simulink model "gm_smartCart4_work"  (R2016a)
settings: Solver=FixedStepDiscrete  StartTime=0.0  StopTime=500000  FixedStep=1  RelTol=1e-3
libraries: simulink x103, hdlsllib x73
(part 2 of 3)

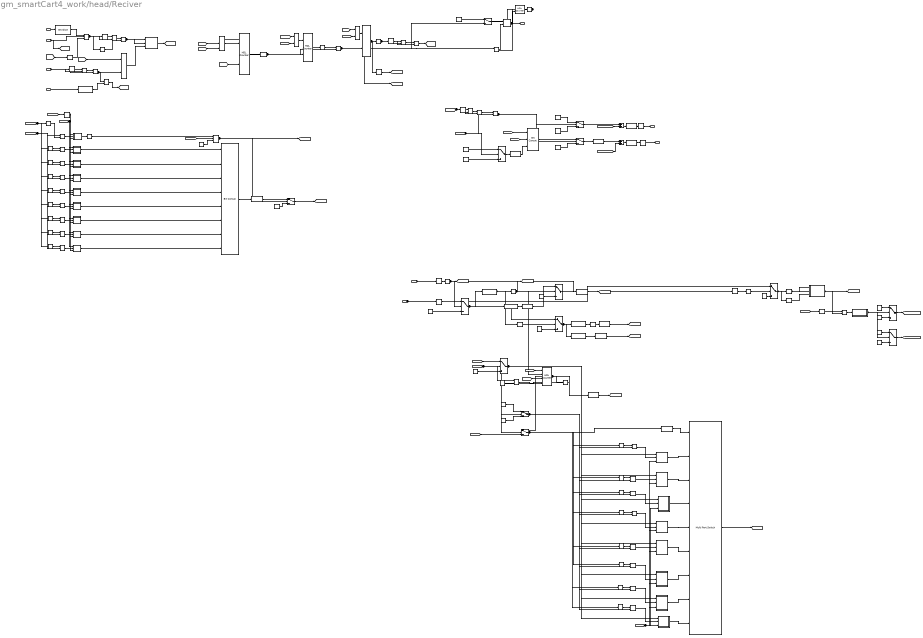
== system gm_smartCart4_work/head/Reciver ==
  note: Схема обнаружение сообщения (1)
  note: cхема управления и синхронизации (2)
  note: Схема формирования отчёта о работе приёмника (4)
  note: Схема связи (5)
  note: Cхема формирования байта и проверка четности
  RST : Inport  OutDataTypeStr=fixdt(1,4,0)  SampleTime=1
  IO : Inport  Port=2  OutDataTypeStr=boolean  SampleTime=1
  STOP : Inport  Port=3  OutDataTypeStr=boolean  SampleTime=1
  adr_IN : Inport  Port=4  OutDataTypeStr=uint8  SampleTime=1
  data_in : Inport  Port=5  OutDataTypeStr=uint32  SampleTime=1
  ON_RECIVER : Inport  Port=6  OutDataTypeStr=boolean  SampleTime=1
  Add : Sum
  Add1 : Sum
  Bit Concat : hdlsllib/HDL Operations/Bit Concat  numInputs=8
  Bit Concat1 : hdlsllib/HDL Operations/Bit Concat  numInputs=3
  Bit Slice1 : hdlsllib/HDL Operations/Bit Slice  lidx=3  ridx=3
  Bit Slice2 : hdlsllib/HDL Operations/Bit Slice  lidx=1  ridx=0
  Bit Slice3 : hdlsllib/HDL Operations/Bit Slice  lidx=7  ridx=2
  Bit Slice4 : hdlsllib/HDL Operations/Bit Slice  lidx=2  ridx=2
  Bit Slice5 : hdlsllib/HDL Operations/Bit Slice  lidx=8  ridx=3
  Compare To Constant{1,3,13,21,31..32} (6 alike) : simulink/Logic and Bit Operations/Compare To Constant  relop===  const=0  OutDataTypeStr=boolean
  Compare To Constant10 : simulink/Logic and Bit Operations/Compare To Constant  relop===  const=7  OutDataTypeStr=boolean
  Compare To Constant11 : simulink/Logic and Bit Operations/Compare To Constant  relop===  const=8  OutDataTypeStr=boolean
  Compare To Constant14 : simulink/Logic and Bit Operations/Compare To Constant  relop===  const=6  OutDataTypeStr=boolean
  Compare To Constant15 : simulink/Logic and Bit Operations/Compare To Constant  relop===  const=7  OutDataTypeStr=boolean
  Compare To Constant{5,16,18,20,22,30} (6 alike) : simulink/Logic and Bit Operations/Compare To Constant  relop===  const=1  OutDataTypeStr=boolean
  Compare To Constant17 : simulink/Logic and Bit Operations/Compare To Constant  relop===  const=200  OutDataTypeStr=boolean
  Compare To Constant19 : simulink/Logic and Bit Operations/Compare To Constant  relop===  const=2  OutDataTypeStr=boolean
  Compare To Constant2 : simulink/Logic and Bit Operations/Compare To Constant  relop===  const=10  OutDataTypeStr=boolean
  Compare To Constant23 : simulink/Logic and Bit Operations/Compare To Constant  relop===  const=2  OutDataTypeStr=boolean
  Compare To Constant24 : simulink/Logic and Bit Operations/Compare To Constant  relop===  const=3  OutDataTypeStr=boolean
  Compare To Constant25 : simulink/Logic and Bit Operations/Compare To Constant  relop===  const=4  OutDataTypeStr=boolean
  Compare To Constant26 : simulink/Logic and Bit Operations/Compare To Constant  relop===  const=5  OutDataTypeStr=boolean
  Compare To Constant27 : simulink/Logic and Bit Operations/Compare To Constant  relop===  const=6  OutDataTypeStr=boolean
  Compare To Constant28 : simulink/Logic and Bit Operations/Compare To Constant  relop===  const=7  OutDataTypeStr=boolean
  Compare To Constant29 : simulink/Logic and Bit Operations/Compare To Constant  relop===  const=5  OutDataTypeStr=boolean
  Compare To Constant4 : simulink/Logic and Bit Operations/Compare To Constant  relop===  const=2604  OutDataTypeStr=boolean
  Compare To Constant6 : simulink/Logic and Bit Operations/Compare To Constant  relop===  const=2  OutDataTypeStr=boolean
  Compare To Constant7 : simulink/Logic and Bit Operations/Compare To Constant  relop===  const=3  OutDataTypeStr=boolean
  Compare To Constant8 : simulink/Logic and Bit Operations/Compare To Constant  relop===  const=4  OutDataTypeStr=boolean
  Compare To Constant9 : simulink/Logic and Bit Operations/Compare To Constant  relop===  const=5  OutDataTypeStr=boolean
  Constant : Constant  Value=0  OutDataTypeStr=uint8
  Constant1 : Constant  Value=0  OutDataTypeStr=uint8
  Constant10 : Constant  Value=0  OutDataTypeStr=boolean  SampleTime=-1
  Constant11 : Constant  Value=0  OutDataTypeStr=boolean
  Constant12 : Constant  Value=0  OutDataTypeStr=uint8
  Constant{3,7,13..15} (5 alike) : Constant  Value=0  OutDataTypeStr=uint32  SampleTime=-1
  Constant16 : Constant  Value=0  OutDataTypeStr=uint8  SampleTime=-1
  Constant17 : Constant  Value=5  OutDataTypeStr=uint8  SampleTime=-1
  Constant18 : Constant  OutDataTypeStr=uint8  SampleTime=-1
  Constant2 : Constant  OutDataTypeStr=uint8
  Constant4 : Constant  Value=2  OutDataTypeStr=fixdt(0,2,0)
  Constant5 : Constant  Value=0  OutDataTypeStr=uint8  SampleTime=-1
  Constant6 : Constant  OutDataTypeStr=boolean
  Constant8 : Constant  OutDataTypeStr=fixdt(0,2,0)
  Constant9 : Constant  OutDataTypeStr=boolean
  Data Type Conversion : DataTypeConversion  OutDataTypeStr=uint8
  Data Type Conversion1 : DataTypeConversion  OutDataTypeStr=fixdt(0,5,0)
  Data Type Conversion10 : DataTypeConversion  OutDataTypeStr=uint8
  Data Type Conversion2 : DataTypeConversion  OutDataTypeStr=uint8
  Data Type Conversion3 : DataTypeConversion  OutDataTypeStr=boolean
  Data Type Conversion4 : DataTypeConversion  OutDataTypeStr=uint32
  Data Type Conversion5 : DataTypeConversion  OutDataTypeStr=uint32
  Data Type Conversion6 : DataTypeConversion  OutDataTypeStr=fixdt(0,5,0)
  Data Type Conversion7 : DataTypeConversion  OutDataTypeStr=fixdt(0,2,0)
  Data Type Conversion8 : DataTypeConversion  OutDataTypeStr=fixdt(1,4,0)
  Data Type Conversion9 : DataTypeConversion  OutDataTypeStr=uint32
  Delay{,1..9,11} (11 alike) : Delay  DelayLength=1  InitialCondition=0
  HDL Counter : hdlsllib/HDL Operations/HDL Counter  CountType=Free running  CountInit=0  CountStep=1  CountMax=1  CountFromType=Initial value  CountFrom=0  CountResetPort=on  CountLoadPort=off  CountEnbPort=on  CountDirPort=off  CountDataType=Unsigned  CountWordLen=13  CountFracLen=0  CountSampTime=1
  HDL Counter1 : hdlsllib/HDL Operations/HDL Counter  CountType=Free running  CountInit=0  CountStep=1  CountMax=1  CountFromType=Initial value  CountFrom=0  CountResetPort=on  CountLoadPort=off  CountEnbPort=on  CountDirPort=off  CountDataType=Unsigned  CountWordLen=1  CountFracLen=0  CountSampTime=1
  HDL Counter2 : hdlsllib/HDL Operations/HDL Counter  CountType=Count limited  CountInit=0  CountStep=1  CountMax=10  CountFromType=Initial value  CountFrom=0  CountResetPort=on  CountLoadPort=off  CountEnbPort=on  CountDirPort=off  CountDataType=Unsigned  CountWordLen=4  CountFracLen=0  CountSampTime=1
  HDL Counter3 : hdlsllib/HDL Operations/HDL Counter  CountType=Free running  CountInit=0  CountStep=1  CountMax=1  CountFromType=Initial value  CountFrom=0  CountResetPort=on  CountLoadPort=on  CountEnbPort=on  CountDirPort=off  CountDataType=Unsigned  CountWordLen=5  CountFracLen=0  CountSampTime=1
  HDL Counter4 : hdlsllib/HDL Operations/HDL Counter  CountType=Free running  CountInit=0  CountStep=1  CountMax=1  CountFromType=Initial value  CountFrom=0  CountResetPort=on  CountLoadPort=off  CountEnbPort=on  CountDirPort=off  CountDataType=Unsigned  CountWordLen=8  CountFracLen=0  CountSampTime=1
  Index Vector : MultiPortSwitch  DataPortOrder=Zero-based contiguous  Inputs=8  zeroidx=on
  Logical Operator{,3,7,9,12..20,33,36,38..46} (24 alike) : Logic  AllPortsSameDT=off  OutDataTypeStr=boolean
  Logical Operator{1,10..11,34..35,48} (6 alike) : Logic  Operator=OR  AllPortsSameDT=off  OutDataTypeStr=boolean
  Logical Operator{2,5..6,32} (4 alike) : Logic  Operator=XOR  AllPortsSameDT=off  OutDataTypeStr=boolean
  Logical Operator22 : Logic  Inputs=3  AllPortsSameDT=off  OutDataTypeStr=boolean
  Logical Operator25 : Logic  Inputs=3  AllPortsSameDT=off  OutDataTypeStr=boolean
  Logical Operator37 : Logic  Operator=NOT  AllPortsSameDT=off  OutDataTypeStr=boolean
  Logical Operator4 : Logic  Operator=NOT  AllPortsSameDT=off  OutDataTypeStr=boolean
  Logical Operator47 : Logic  Operator=NOT  Inputs=3  AllPortsSameDT=off  OutDataTypeStr=boolean
  Logical Operator8 : Logic  Operator=OR  Inputs=3  AllPortsSameDT=off  OutDataTypeStr=boolean
  SA12 : simulink/Additional Math & Discrete/Additional Discrete/Unit Delay Enabled  vinit=0  tsamp=-1
  Switch{1..14} (14 alike) : Switch  Criteria=u2 ~= 0
  Unit Delay Enabled Resettable : Subsystem
  Unit Delay Enabled Resettable1 : Subsystem
  Unit Delay Enabled Resettable11 : Subsystem
  Unit Delay Enabled Resettable12 : Subsystem
  Unit Delay Enabled Resettable13 : Subsystem
  Unit Delay Enabled Resettable14 : Subsystem
  Unit Delay Enabled Resettable15 : Subsystem
  Unit Delay Enabled Resettable16 : Subsystem
  Unit Delay Enabled Resettable17 : Subsystem
  Unit Delay Enabled Resettable18 : Subsystem
  Unit Delay Enabled Resettable19 : Subsystem
  Unit Delay Enabled Resettable2 : Subsystem
  Unit Delay Enabled Resettable3 : Subsystem
  Unit Delay Enabled Resettable4 : Subsystem
  Unit Delay Enabled Resettable5 : Subsystem
  Unit Delay Enabled Resettable6 : Subsystem
  Unit Delay Enabled Resettable7 : Subsystem
  Unit Delay Enabled Resettable8 : Subsystem
  Unit Delay Enabled Resettable9 : Subsystem
  signal_edg : Subsystem
  signal_edg5 : Subsystem
  AddrOUT : Outport  OutDataTypeStr=uint8
  STATUS : Outport  Port=2  OutDataTypeStr=uint32
  Strob : Outport  Port=3  OutDataTypeStr=boolean
  wires:
  RST/1 -> Bit Slice1/1
  IO/1 -> Logical Operator25/2, [data]
  STOP/1 -> Logical Operator9/2, Logical Operator5/2, Delay1/1
  adr_IN/1 -> Delay9/1, Delay7/1
  data_in/1 -> Switch12/1, Delay11/1
  ON_RECIVER/1 -> signal_edg5/1(In1)
  Add/1 -> Data Type Conversion9/1
  Add1/1 -> Data Type Conversion10/1
  Bit Concat/1 -> Data Type Conversion/1
  Bit Concat1/1 -> Switch3/1
  Bit Slice1/1 -> Logical Operator25/1
  Bit Slice2/1 -> Compare To Constant19/1, Compare To Constant18/1
  Bit Slice3/1 -> Data Type Conversion5/1
  Bit Slice4/1 -> Compare To Constant20/1
  Bit Slice5/1 -> Data Type Conversion1/1
  Compare To Constant1/1 -> Logical Operator/1
  Compare To Constant10/1 -> Logical Operator19/1
  Compare To Constant11/1 -> Logical Operator20/1
  Compare To Constant13/1 -> Logical Operator22/1
  Compare To Constant14/1 -> Logical Operator18/1
  Compare To Constant15/1 -> Logical Operator37/1
  Compare To Constant16/1 -> Switch11/2, [Send_com]
  Compare To Constant17/1 -> Switch8/2, Logical Operator34/2, HDL Counter4/1
  Compare To Constant18/1 -> Switch7/2, HDL Counter3/2, [WE]
  Compare To Constant19/1 -> Switch9/2
  Compare To Constant2/1 -> Logical Operator7/2, Logical Operator6/2, Delay2/1
  Compare To Constant20/1 -> Data Type Conversion3/1
  Compare To Constant21/1 -> Logical Operator39/1
  Compare To Constant22/1 -> Logical Operator40/1
  Compare To Constant23/1 -> Logical Operator41/1
  Compare To Constant24/1 -> Logical Operator42/1
  Compare To Constant25/1 -> Logical Operator43/1
  Compare To Constant26/1 -> Logical Operator44/1
  Compare To Constant27/1 -> Logical Operator45/1
  Compare To Constant28/1 -> Logical Operator46/1
  Compare To Constant29/1 -> Switch12/2
  Compare To Constant3/1 -> Logical Operator12/2
  Compare To Constant30/1 -> Unit Delay Enabled Resettable17/2(Enb), Unit Delay Enabled Resettable17/1(data_in)
  Compare To Constant31/1 -> Logical Operator38/1
  Compare To Constant32/1 -> Unit Delay Enabled Resettable17/3(Reset)
  Compare To Constant4/1 -> Logical Operator8/1, Logical Operator/2, HDL Counter1/2
  Compare To Constant5/1 -> Logical Operator13/1
  Compare To Constant6/1 -> Logical Operator14/1
  Compare To Constant7/1 -> Logical Operator15/1
  Compare To Constant8/1 -> Logical Operator16/1
  Compare To Constant9/1 -> Logical Operator17/1
  Constant/1 -> Switch1/3
  Constant1/1 -> Switch2/3
  Constant10/1 -> Switch8/1
  Constant11/1 -> Switch5/3
  Constant12/1 -> Switch3/3
  Constant13/1 -> Switch12/3
  Constant14/1 -> Switch11/3
  Constant15/1 -> Switch14/3
  Constant16/1 -> Switch13/3
  Constant17/1 -> Switch13/1
  Constant18/1 -> Switch14/1
  Constant2/1 -> Switch2/1
  Constant3/1 -> Switch7/3
  Constant4/1 -> Switch10/1
  Constant5/1 -> Switch4/3
  Constant6/1 -> Switch5/1
  Constant7/1 -> Switch9/3
  Constant8/1 -> Switch10/3
  Constant9/1 -> Logical Operator22/3
  Data Type Conversion/1 -> Switch1/1
  Data Type Conversion1/1 -> [addRd]
  Data Type Conversion10/1 -> Delay8/1
  Data Type Conversion2/1 -> [Num_Count]
  Data Type Conversion3/1 -> [RD]
  Data Type Conversion4/1 -> Add/1
  Data Type Conversion5/1 -> Switch7/1
  Data Type Conversion6/1 -> [VAL_COUNT]
  Data Type Conversion7/1 -> Bit Concat1/3
  Data Type Conversion8/1 -> Index Vector/1
  Data Type Conversion9/1 -> Delay6/1
  Delay/1 -> Logical Operator2/1
  Delay1/1 -> Logical Operator5/1
  Delay11/1 -> Switch11/1
  Delay2/1 -> Logical Operator6/1
  Delay3/1 -> [Number_bit]
  Delay4/1 -> Logical Operator32/1
  Delay5/1 -> Unit Delay Enabled Resettable9/3(Reset), Unit Delay Enabled Resettable8/3(Reset), Unit Delay Enabled Resettable7/3(Reset), Unit Delay Enabled Resettable6/3(Reset), Unit Delay Enabled Resettable5/3(Reset), Unit Delay Enabled Resettable4/3(Reset), Unit Delay Enabled Resettable3/3(Reset), Unit Delay Enabled Resettable2/3(Reset), Unit Delay Enabled Resettable1/3(Reset)
  Delay6/1 -> STATUS/1
  Delay7/1 -> Compare To Constant16/1
  Delay8/1 -> AddrOUT/1
  Delay9/1 -> Compare To Constant29/1
  [bait_done] -> Logical Operator1/1
  [data] -> Unit Delay Enabled Resettable9/1(data_in), Unit Delay Enabled Resettable8/1(data_in), Unit Delay Enabled Resettable7/1(data_in), Unit Delay Enabled Resettable6/1(data_in), Unit Delay Enabled Resettable5/1(data_in), Unit Delay Enabled Resettable4/1(data_in), Unit Delay Enabled Resettable3/1(data_in), Unit Delay Enabled Resettable2/1(data_in), Unit Delay Enabled Resettable1/1(data_in)
  [data] -> Compare To Constant31/1
  [detect_error] -> Logical Operator47/1
  [Mes_res] -> HDL Counter/2
  [bait_done] -> Logical Operator22/2
  [Error_bait] -> Logical Operator33/2, Logical Operator32/2, Delay4/1
  [Error_bait] -> Switch6/2, Switch5/2, Switch4/2, Logical Operator36/1
  [bait] -> Switch4/1
  [Num_Count] -> Bit Concat1/2
  [bait_done] -> Delay5/1
  [Read_Byte] -> Bit Concat1/1
  [RST] -> Unit Delay Enabled Resettable19/3(Reset), Unit Delay Enabled Resettable18/3(Reset), Unit Delay Enabled Resettable16/3(Reset), Unit Delay Enabled Resettable15/3(Reset), Unit Delay Enabled Resettable14/3(Reset), Unit Delay Enabled Resettable13/3(Reset), Unit Delay Enabled Resettable12/3(Reset), Unit Delay Enabled Resettable11/3(Reset)
  [VAL_COUNT] -> HDL Counter3/3
  [RD] -> Switch10/2, Logical Operator35/2
  [bait_done] -> Logical Operator10/1
  [addRd] -> Switch6/3
  [data_detect_error] -> Add/2
  [addr_detect_error] -> Add1/2
  [RST] -> HDL Counter3/1
  [bait_done] -> Logical Operator11/1
  [bait_done] -> Logical Operator8/2
  [RST] -> Logical Operator8/3
  [RST] -> Logical Operator10/2
  [RST] -> Logical Operator11/2
  [Get_val] -> Logical Operator20/2, Logical Operator19/2, Logical Operator18/2, Logical Operator17/2, Logical Operator16/2, Logical Operator15/2, Logical Operator14/2, Logical Operator13/2, Logical Operator12/1
  [Number_bit] -> Compare To Constant9/1, Compare To Constant8/1, Compare To Constant7/1, Compare To Constant6/1, Compare To Constant5/1, Compare To Constant3/1, Compare To Constant14/1, Compare To Constant11/1, Compare To Constant10/1
  HDL Counter/1 -> Compare To Constant4/1
  HDL Counter1/1 -> Compare To Constant1/1
  HDL Counter2/1 -> Compare To Constant2/1, Delay3/1
  HDL Counter3/1 -> Switch6/1, Data Type Conversion2/1, Compare To Constant15/1
  HDL Counter4/1 -> Compare To Constant17/1
  Index Vector/1 -> [Read_Byte]
  Logical Operator/1 -> Switch8/3, Logical Operator34/1, HDL Counter2/2, [Get_val]
  Logical Operator1/1 -> Unit Delay Enabled Resettable/3(Reset)
  Logical Operator10/1 -> HDL Counter1/1
  Logical Operator11/1 -> HDL Counter2/1
  Logical Operator12/1 -> Unit Delay Enabled Resettable1/2(Enb)
  Logical Operator13/1 -> Unit Delay Enabled Resettable2/2(Enb)
  Logical Operator14/1 -> Unit Delay Enabled Resettable3/2(Enb)
  Logical Operator15/1 -> Unit Delay Enabled Resettable4/2(Enb)
  Logical Operator16/1 -> Unit Delay Enabled Resettable5/2(Enb)
  Logical Operator17/1 -> Unit Delay Enabled Resettable6/2(Enb)
  Logical Operator18/1 -> Unit Delay Enabled Resettable7/2(Enb)
  Logical Operator19/1 -> Unit Delay Enabled Resettable8/2(Enb)
  Logical Operator2/1 -> Logical Operator3/1
  Logical Operator20/1 -> Unit Delay Enabled Resettable9/2(Enb)
  Logical Operator22/1 -> Switch1/2, [Error_bait]
  Logical Operator25/1 -> Logical Operator4/1, Logical Operator2/2, Delay/1
  Logical Operator3/1 -> Unit Delay Enabled Resettable/2(Enb), Unit Delay Enabled Resettable/1(data_in)
  Logical Operator32/1 -> Logical Operator33/1
  Logical Operator33/1 -> Logical Operator35/1
  Logical Operator34/1 -> SA12/2
  Logical Operator35/1 -> Switch3/2, Switch2/2
  Logical Operator36/1 -> HDL Counter3/4
  Logical Operator37/1 -> Logical Operator36/2
  Logical Operator38/1 -> signal_edg/1(In1)
  Logical Operator39/1 -> Unit Delay Enabled Resettable11/2(Enb)
  Logical Operator4/1 -> Logical Operator3/2
  Logical Operator40/1 -> Unit Delay Enabled Resettable12/2(Enb)
  Logical Operator41/1 -> Unit Delay Enabled Resettable13/2(Enb)
  Logical Operator42/1 -> Unit Delay Enabled Resettable14/2(Enb)
  Logical Operator43/1 -> Unit Delay Enabled Resettable15/2(Enb)
  Logical Operator44/1 -> Unit Delay Enabled Resettable16/2(Enb)
  Logical Operator45/1 -> Unit Delay Enabled Resettable18/2(Enb)
  Logical Operator46/1 -> Unit Delay Enabled Resettable19/2(Enb)
  Logical Operator47/1 -> Logical Operator25/3
  Logical Operator48/1 -> [RST]
  Logical Operator5/1 -> Logical Operator9/1
  Logical Operator6/1 -> Logical Operator7/1
  Logical Operator7/1 -> [bait_done]
  Logical Operator8/1 -> HDL Counter/1
  Logical Operator9/1 -> Logical Operator48/1, Logical Operator1/2
  SA12/1 -> HDL Counter4/2, Strob/1
  Switch1/1 -> [bait]
  Switch10/1 -> Data Type Conversion7/1
  Switch11/1 -> Switch9/1, Bit Slice3/1, Bit Slice2/1
  Switch12/1 -> Compare To Constant32/1, Compare To Constant30/1
  Switch13/1 -> [addr_detect_error]
  Switch14/1 -> [data_detect_error]
  Switch2/1 -> Add1/1
  Switch3/1 -> Data Type Conversion4/1
  Switch4/1 -> Unit Delay Enabled Resettable19/1(data_in), Unit Delay Enabled Resettable18/1(data_in), Unit Delay Enabled Resettable16/1(data_in), Unit Delay Enabled Resettable15/1(data_in), Unit Delay Enabled Resettable14/1(data_in), Unit Delay Enabled Resettable13/1(data_in), Unit Delay Enabled Resettable12/1(data_in), Unit Delay Enabled Resettable11/1(data_in)
  Switch5/1 -> Logical Operator46/2, Logical Operator45/2, Logical Operator44/2, Logical Operator43/2, Logical Operator42/2, Logical Operator41/2, Logical Operator40/2, Logical Operator39/2
  Switch6/1 -> Data Type Conversion8/1, Compare To Constant28/1, Compare To Constant27/1, Compare To Constant26/1, Compare To Constant25/1, Compare To Constant24/1, Compare To Constant23/1, Compare To Constant22/1, Compare To Constant21/1
  Switch7/1 -> Data Type Conversion6/1
  Switch8/1 -> SA12/1
  Switch9/1 -> Bit Slice5/1, Bit Slice4/1
  Unit Delay Enabled Resettable/1(data_out) -> [Mes_res]
  Unit Delay Enabled Resettable1/1(data_out) -> Compare To Constant13/1
  Unit Delay Enabled Resettable11/1(data_out) -> Index Vector/2
  Unit Delay Enabled Resettable12/1(data_out) -> Index Vector/3
  Unit Delay Enabled Resettable13/1(data_out) -> Index Vector/4
  Unit Delay Enabled Resettable14/1(data_out) -> Index Vector/5
  Unit Delay Enabled Resettable15/1(data_out) -> Index Vector/6
  Unit Delay Enabled Resettable16/1(data_out) -> Index Vector/7
  Unit Delay Enabled Resettable17/1(data_out) -> Logical Operator38/2, [detect_error]
  Unit Delay Enabled Resettable18/1(data_out) -> Index Vector/8
  Unit Delay Enabled Resettable19/1(data_out) -> Index Vector/9
  Unit Delay Enabled Resettable2/1(data_out) -> Bit Concat/1
  Unit Delay Enabled Resettable3/1(data_out) -> Bit Concat/2
  Unit Delay Enabled Resettable4/1(data_out) -> Bit Concat/3
  Unit Delay Enabled Resettable5/1(data_out) -> Bit Concat/4
  Unit Delay Enabled Resettable6/1(data_out) -> Bit Concat/5
  Unit Delay Enabled Resettable7/1(data_out) -> Bit Concat/6
  Unit Delay Enabled Resettable8/1(data_out) -> Bit Concat/7
  Unit Delay Enabled Resettable9/1(data_out) -> Bit Concat/8
  signal_edg/1(Out1) -> Switch14/2, Switch13/2
  signal_edg5/1(Out1) -> Logical Operator48/2

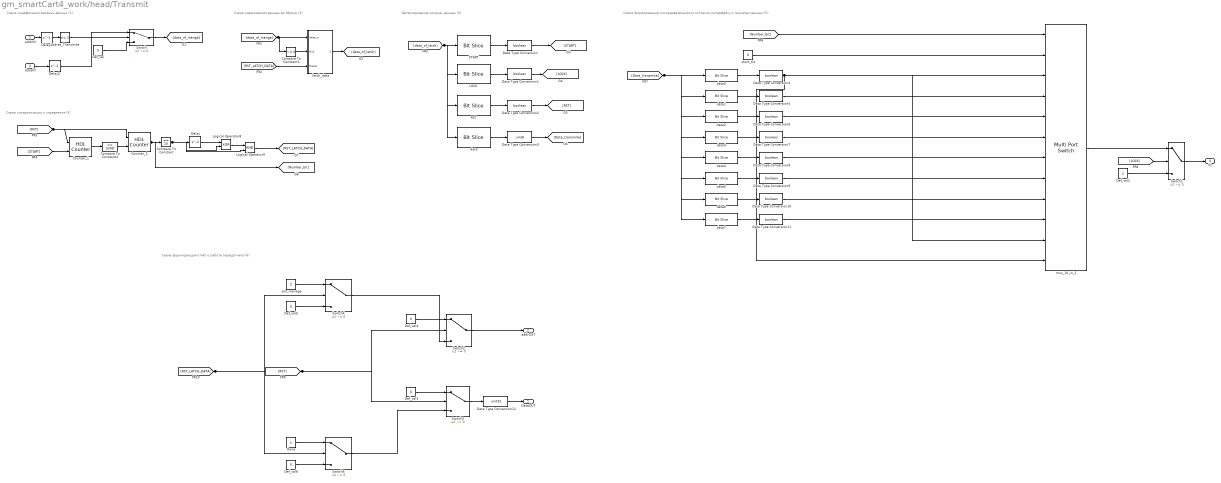
== system gm_smartCart4_work/head/Transmit ==
  note: Схема синхронизации и управления (4)
  note: Схема индефикации входных данных (1)
  note: Схема удерживания данных до сброса (2)
  note: Детектирование команд, данных (3)
  note: Схема формирование последовательности согласно интерфейсу и принятых данных (5)
  note: Схема формирующая отчёт о работе передатчика (6)
  addrIN : Inport  OutDataTypeStr=uint8  SampleTime=1
  dataIN : Inport  Port=2  OutDataTypeStr=fixdt(0,32,0)  SampleTime=1
  Compare To Constant : simulink/Logic and Bit Operations/Compare To Constant  relop===  const=10  OutDataTypeStr=boolean
  Compare To Constant1 : simulink/Logic and Bit Operations/Compare To Constant  relop=~=  const=0  OutDataTypeStr=boolean
  Compare To Constant2 : simulink/Logic and Bit Operations/Compare To Constant  relop===  const=5208  OutDataTypeStr=boolean
  Counter_1 : hdlsllib/HDL Operations/HDL Counter  CountType=Count limited  CountInit=0  CountStep=1  CountMax=5208  CountFromType=Initial value  CountFrom=0  CountResetPort=on  CountLoadPort=off  CountEnbPort=on  CountDirPort=off  CountDataType=Unsigned  CountWordLen=13  CountFracLen=0  CountSampTime=1
  Counter_2 : hdlsllib/HDL Operations/HDL Counter  CountType=Count limited  CountInit=0  CountStep=1  CountMax=11  CountFromType=Initial value  CountFrom=0  CountResetPort=on  CountLoadPort=off  CountEnbPort=on  CountDirPort=off  CountDataType=Unsigned  CountWordLen=4  CountFracLen=0  CountSampTime=1
  Data Type Conversion{,1..2,4..11} (11 alike) : DataTypeConversion  OutDataTypeStr=boolean
  Data Type Conversion12 : DataTypeConversion  OutDataTypeStr=uint32
  Data Type Conversion3 : DataTypeConversion  OutDataTypeStr=uint8
  Def_val : Constant  Value=0  OutDataTypeStr=fixdt(0,32,0)  SampleTime=-1
  Def_val2 : Constant  OutDataTypeStr=boolean  SampleTime=-1
  Def_val{3..6} (4 alike) : Constant  Value=0  OutDataTypeStr=uint8  SampleTime=-1
  Delay : Delay
  Delay1 : Delay  DelayLength=1  InitialCondition=0
  Delay2 : Delay  DelayLength=1  InitialCondition=0
  Done : Constant  OutDataTypeStr=uint8  SampleTime=-1
  LOCK : hdlsllib/HDL Operations/Bit Slice  lidx=1  ridx=1
  Logical Operator8 : Logic  Operator=XOR  AllPortsSameDT=off  OutDataTypeStr=boolean
  Logical Operator9 : Logic  AllPortsSameDT=off  OutDataTypeStr=boolean
  RST : hdlsllib/HDL Operations/Bit Slice  lidx=2  ridx=2
  START : hdlsllib/HDL Operations/Bit Slice  lidx=0  ridx=0
  Switch{,1..5} (6 alike) : Switch  Criteria=u2 ~= 0
  adr_manage : Constant  Value=2  OutDataTypeStr=uint8  SampleTime=-1
  adres_Transmite : simulink/Logic and Bit Operations/Compare To Constant  relop===  const=2  OutDataTypeStr=boolean
  data : hdlsllib/HDL Operations/Bit Slice  lidx=10  ridx=3
  "data0 " : hdlsllib/HDL Operations/Bit Slice  lidx=0  ridx=0
  data1 : hdlsllib/HDL Operations/Bit Slice  lidx=1  ridx=1
  data2 : hdlsllib/HDL Operations/Bit Slice  lidx=2  ridx=2
  data3 : hdlsllib/HDL Operations/Bit Slice  lidx=3  ridx=3
  data4 : hdlsllib/HDL Operations/Bit Slice  lidx=4  ridx=4
  data5 : hdlsllib/HDL Operations/Bit Slice  lidx=5  ridx=5
  data6 : hdlsllib/HDL Operations/Bit Slice  lidx=6  ridx=6
  data7 : hdlsllib/HDL Operations/Bit Slice  lidx=7  ridx=7
  latch_data : Subsystem
  mux_10_in_1 : MultiPortSwitch  DataPortOrder=Zero-based contiguous  Inputs=11  zeroidx=on
  start_bit : Constant  Value=0  OutDataTypeStr=boolean  SampleTime=-1
  DataOUT : Outport  OutDataTypeStr=uint32
  addrOUT : Outport  Port=2  OutDataTypeStr=uint8
  IO : Outport  Port=3  OutDataTypeStr=boolean
  wires:
  addrIN/1 -> Delay1/1
  dataIN/1 -> Delay2/1
  Compare To Constant/1 -> Logical Operator9/2, Logical Operator8/2, Delay/1
  Compare To Constant1/1 -> latch_data/2(Enb)
  Compare To Constant2/1 -> Counter_2/2
  Counter_1/1 -> Compare To Constant2/1
  Counter_2/1 -> Compare To Constant/1, [Number_bit]
  Data Type Conversion/1 -> [START]
  Data Type Conversion1/1 -> [LOCK]
  Data Type Conversion10/1 -> mux_10_in_1/9
  Data Type Conversion11/1 -> mux_10_in_1/10
  Data Type Conversion12/1 -> DataOUT/1
  Data Type Conversion2/1 -> [RST]
  Data Type Conversion3/1 -> [Data_transmite]
  Data Type Conversion4/1 -> mux_10_in_1/12, mux_10_in_1/11, mux_10_in_1/3
  Data Type Conversion5/1 -> mux_10_in_1/4
  Data Type Conversion6/1 -> mux_10_in_1/5
  Data Type Conversion7/1 -> mux_10_in_1/6
  Data Type Conversion8/1 -> mux_10_in_1/7
  Data Type Conversion9/1 -> mux_10_in_1/8
  Def_val/1 -> Switch/3
  Def_val2/1 -> Switch1/3
  Def_val3/1 -> Switch3/1
  Def_val4/1 -> Switch2/1
  Def_val5/1 -> Switch4/3
  Def_val6/1 -> Switch5/3
  Delay/1 -> Logical Operator8/1
  Delay1/1 -> adres_Transmite/1
  Delay2/1 -> Switch/1
  Done/1 -> Switch5/1
  [data_of_mange] -> Compare To Constant1/1, latch_data/1(data_in)
  [RST_LATCH_DATA] -> Switch5/2, Switch4/2
  [RST_LATCH_DATA] -> latch_data/3(Reset)
  [data_of_latch] -> data/1, START/1, RST/1, LOCK/1
  [START] -> Counter_1/2
  [RST] -> Counter_2/1, Counter_1/1
  [Number_bit] -> mux_10_in_1/1
  [Data_transmite] -> data7/1, data6/1, data5/1, data4/1, data3/1, data2/1, data1/1, "data0 "/1
  [LOCK] -> Switch1/2
  [RST] -> Switch3/2, Switch2/2
  LOCK/1 -> Data Type Conversion1/1
  Logical Operator8/1 -> Logical Operator9/1
  Logical Operator9/1 -> [RST_LATCH_DATA]
  RST/1 -> Data Type Conversion2/1
  START/1 -> Data Type Conversion/1
  Switch/1 -> [data_of_mange]
  Switch1/1 -> IO/1
  Switch2/1 -> addrOUT/1
  Switch3/1 -> Data Type Conversion12/1
  Switch4/1 -> Switch2/3
  Switch5/1 -> Switch3/3
  adr_manage/1 -> Switch4/1
  adres_Transmite/1 -> Switch/2
  data/1 -> Data Type Conversion3/1
  "data0 "/1 -> Data Type Conversion4/1
  data1/1 -> Data Type Conversion5/1
  data2/1 -> Data Type Conversion6/1
  data3/1 -> Data Type Conversion7/1
  data4/1 -> Data Type Conversion8/1
  data5/1 -> Data Type Conversion9/1
  data6/1 -> Data Type Conversion10/1
  data7/1 -> Data Type Conversion11/1
  latch_data/1(data_out) -> [data_of_latch]
  mux_10_in_1/1 -> Switch1/1
  start_bit/1 -> mux_10_in_1/2

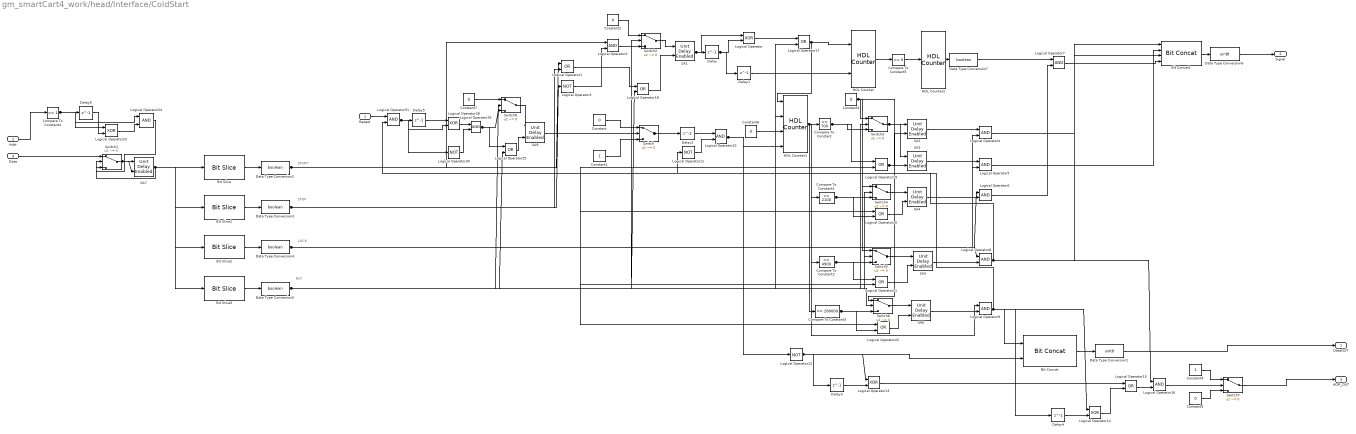
== system gm_smartCart4_work/head/Interface/ColdStart ==
  note: LOCK
  note: STOP
  note: START
  note: RST
  Reqest : Inport  OutDataTypeStr=boolean  SampleTime=1
  Addr : Inport  Port=2  OutDataTypeStr=uint8  SampleTime=1
  Data : Inport  Port=3  OutDataTypeStr=uint8  SampleTime=1
  Bit Concat : hdlsllib/HDL Operations/Bit Concat  numInputs=2
  Bit Concat1 : hdlsllib/HDL Operations/Bit Concat  numInputs=4
  Bit Slice : hdlsllib/HDL Operations/Bit Slice  lidx=3  ridx=3
  Bit Slice1 : hdlsllib/HDL Operations/Bit Slice  lidx=2  ridx=2
  Bit Slice2 : hdlsllib/HDL Operations/Bit Slice  lidx=1  ridx=1
  Bit Slice3 : hdlsllib/HDL Operations/Bit Slice  lidx=0  ridx=0
  Compare To Constant : simulink/Logic and Bit Operations/Compare To Constant  relop===  const=700  OutDataTypeStr=boolean
  Compare To Constant1 : simulink/Logic and Bit Operations/Compare To Constant  relop===  const=2100  OutDataTypeStr=boolean
  Compare To Constant2 : simulink/Logic and Bit Operations/Compare To Constant  relop===  const=4900  OutDataTypeStr=boolean
  Compare To Constant3 : simulink/Logic and Bit Operations/Compare To Constant  relop===  const=280000  OutDataTypeStr=boolean
  Compare To Constant4 : simulink/Logic and Bit Operations/Compare To Constant  relop===  const=1  OutDataTypeStr=boolean
  Compare To Constant5 : simulink/Logic and Bit Operations/Compare To Constant  relop===  const=0  OutDataTypeStr=boolean
  Constant{,2..3,7} (4 alike) : Constant  Value=0  OutDataTypeStr=boolean
  Constant1 : Constant  OutDataTypeStr=boolean
  Constant4 : Constant  OutDataTypeStr=uint8
  Constant5 : Constant  Value=0  OutDataTypeStr=uint8
  Constant6 : Constant  Value=0  OutDataTypeStr=fixdt(0,32,0)
  Data Type Conversion1 : DataTypeConversion  OutDataTypeStr=uint8
  Data Type Conversion{2..5,7} (5 alike) : DataTypeConversion  OutDataTypeStr=boolean
  Data Type Conversion6 : DataTypeConversion  OutDataTypeStr=uint8
  Delay{,1,3..6} (6 alike) : Delay  DelayLength=1  InitialCondition=0
  Delay2 : Delay  InitialCondition=0
  HDL Counter : hdlsllib/HDL Operations/HDL Counter  CountType=Count limited  CountInit=0  CountStep=1  CountMax=6  CountFromType=Initial value  CountFrom=0  CountResetPort=on  CountLoadPort=off  CountEnbPort=on  CountDirPort=off  CountDataType=Unsigned  CountWordLen=3  CountFracLen=0  CountSampTime=277e-9
  HDL Counter1 : hdlsllib/HDL Operations/HDL Counter  CountType=Count limited  CountInit=0  CountStep=1  CountMax=40000  CountFromType=Initial value  CountFrom=0  CountResetPort=on  CountLoadPort=on  CountEnbPort=on  CountDirPort=off  CountDataType=Unsigned  CountWordLen=32  CountFracLen=0  CountSampTime=277e-9
  HDL Counter2 : hdlsllib/HDL Operations/HDL Counter  CountType=Free running  CountInit=0  CountStep=1  CountMax=5  CountFromType=Initial value  CountFrom=0  CountResetPort=off  CountLoadPort=off  CountEnbPort=on  CountDirPort=off  CountDataType=Unsigned  CountWordLen=1  CountFracLen=0  CountSampTime=277e-9
  Logical Operator{,13..14,23,28} (5 alike) : Logic  Operator=XOR  AllPortsSameDT=off  OutDataTypeStr=boolean
  Logical Operator{1,15,17..22,25} (9 alike) : Logic  Operator=OR  AllPortsSameDT=off  OutDataTypeStr=boolean
  Logical Operator{2,4..10,16,24,29,31} (12 alike) : Logic  AllPortsSameDT=off  OutDataTypeStr=boolean
  Logical Operator{3,11..12,30} (4 alike) : Logic  Operator=NOT  AllPortsSameDT=off  OutDataTypeStr=boolean
  SA{1..7,9} (8 alike) : simulink/Additional Math & Discrete/Additional Discrete/Unit Delay Enabled  vinit=0  tsamp=-1
  Switch{,1..8} (9 alike) : Switch  Criteria=u2 ~= 0
  DataOUT : Outport  OutDataTypeStr=uint8
  Signal : Outport  Port=2  OutDataTypeStr=uint8
  ADR_OUT : Outport  Port=3  OutDataTypeStr=uint8
  wires:
  Reqest/1 -> Logical Operator31/1
  Addr/1 -> Compare To Constant4/1
  Data/1 -> Switch1/1
  Bit Concat/1 -> Data Type Conversion1/1
  Bit Concat1/1 -> Data Type Conversion6/1
  Bit Slice/1 -> Data Type Conversion2/1
  Bit Slice1/1 -> Data Type Conversion3/1
  Bit Slice2/1 -> Data Type Conversion4/1
  Bit Slice3/1 -> Data Type Conversion5/1
  Compare To Constant/1 -> Switch3/3, Logical Operator19/1
  Compare To Constant1/1 -> Switch4/3, Logical Operator20/2
  Compare To Constant2/1 -> Switch5/3, Logical Operator21/1
  Compare To Constant3/1 -> Switch6/3, Logical Operator22/2
  Compare To Constant4/1 -> Logical Operator24/1, Logical Operator23/1, Delay6/1
  Compare To Constant5/1 -> HDL Counter2/1
  Constant/1 -> Switch/1
  Constant1/1 -> Switch/3
  Constant2/1 -> Switch2/1
  Constant3/1 -> Switch6/1, Switch5/1, Switch4/1, Switch3/1
  Constant4/1 -> Switch7/1
  Constant5/1 -> Switch7/3
  Constant6/1 -> HDL Counter1/3
  Constant7/1 -> Switch8/1
  Data Type Conversion1/1 -> DataOUT/1
  Data Type Conversion2/1 -> Logical Operator2/1, Logical Operator1/1
  Data Type Conversion3/1 -> Logical Operator3/1, Logical Operator1/2
  Data Type Conversion4/1 -> Logical Operator9/1, Logical Operator8/1, Logical Operator6/1, Logical Operator5/2, Logical Operator4/2
  Data Type Conversion5/1 -> Switch8/2, Switch6/2, Switch5/2, Switch4/2, Switch3/2, Switch2/2, Logical Operator25/2, Logical Operator22/1, Logical Operator21/2, Logical Operator20/1, Logical Operator19/2, Logical Operator18/2, Logical Operator17/2, HDL Counter1/2
  Data Type Conversion6/1 -> Signal/1
  Data Type Conversion7/1 -> Logical Operator7/1
  Delay/1 -> Logical Operator/2, Delay1/1
  Delay1/1 -> HDL Counter/2
  Delay2/1 -> Logical Operator10/1
  Delay3/1 -> Logical Operator13/2
  Delay4/1 -> Logical Operator14/2
  Delay5/1 -> Logical Operator28/1
  Delay6/1 -> Logical Operator23/2
  HDL Counter/1 -> Compare To Constant5/1
  HDL Counter1/1 -> Compare To Constant3/1, Compare To Constant2/1, Compare To Constant1/1, Compare To Constant/1
  HDL Counter2/1 -> Data Type Conversion7/1
  Logical Operator/1 -> Logical Operator17/1
  Logical Operator1/1 -> Logical Operator18/1
  Logical Operator10/1 -> Logical Operator12/1, HDL Counter1/4
  Logical Operator11/1 -> Logical Operator10/2
  Logical Operator12/1 -> Logical Operator13/1, Bit Concat/2, Delay3/1
  Logical Operator13/1 -> Logical Operator15/1
  Logical Operator14/1 -> Logical Operator15/2
  Logical Operator15/1 -> Logical Operator16/2
  Logical Operator16/1 -> Switch7/2
  Logical Operator17/1 -> HDL Counter1/1, HDL Counter/1
  Logical Operator18/1 -> SA1/2
  Logical Operator19/1 -> SA3/2, SA2/2
  Logical Operator2/1 -> Switch2/3
  Logical Operator20/1 -> SA4/2
  Logical Operator21/1 -> SA5/2
  Logical Operator22/1 -> SA6/2
  Logical Operator23/1 -> Logical Operator24/2
  Logical Operator24/1 -> Switch1/2
  Logical Operator25/1 -> SA9/2
  Logical Operator28/1 -> Logical Operator29/1
  Logical Operator29/1 -> Switch8/3, Logical Operator25/1
  Logical Operator3/1 -> Logical Operator2/2
  Logical Operator30/1 -> Logical Operator29/2
  Logical Operator31/1 -> Logical Operator30/1, Logical Operator28/2, Delay5/1
  Logical Operator4/1 -> Bit Concat1/3
  Logical Operator5/1 -> Bit Concat1/2
  Logical Operator6/1 -> Logical Operator7/2
  Logical Operator7/1 -> Bit Concat1/4
  Logical Operator8/1 -> Logical Operator31/2, Logical Operator16/1, Bit Concat1/1
  Logical Operator9/1 -> Logical Operator14/1, Logical Operator11/1, Bit Concat/1, Delay4/1
  SA1/1 -> Logical Operator/1, Delay/1
  SA2/1 -> Logical Operator4/1
  SA3/1 -> Logical Operator5/1
  SA4/1 -> Logical Operator6/2
  SA5/1 -> Logical Operator8/2
  SA6/1 -> Logical Operator9/2
  SA7/1 -> Switch1/3, Bit Slice3/1, Bit Slice2/1, Bit Slice1/1, Bit Slice/1
  SA9/1 -> Switch/2
  Switch/1 -> Delay2/1
  Switch1/1 -> SA7/2, SA7/1
  Switch2/1 -> SA1/1
  Switch3/1 -> SA3/1, SA2/1
  Switch4/1 -> SA4/1
  Switch5/1 -> SA5/1
  Switch6/1 -> SA6/1
  Switch7/1 -> ADR_OUT/1
  Switch8/1 -> SA9/1

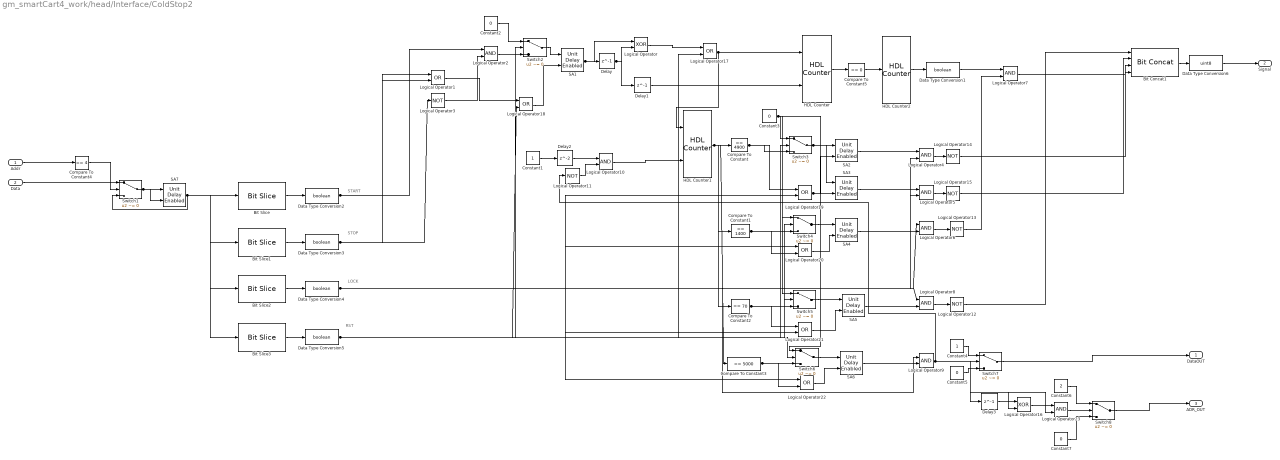
== system gm_smartCart4_work/head/Interface/ColdStop2 ==
  note: LOCK
  note: STOP
  note: START
  note: RST
  Addr : Inport  OutDataTypeStr=uint8  SampleTime=1
  Data : Inport  Port=2  OutDataTypeStr=uint8  SampleTime=1
  Bit Concat1 : hdlsllib/HDL Operations/Bit Concat  numInputs=4
  Bit Slice : hdlsllib/HDL Operations/Bit Slice  lidx=3  ridx=3
  Bit Slice1 : hdlsllib/HDL Operations/Bit Slice  lidx=2  ridx=2
  Bit Slice2 : hdlsllib/HDL Operations/Bit Slice  lidx=1  ridx=1
  Bit Slice3 : hdlsllib/HDL Operations/Bit Slice  lidx=0  ridx=0
  Compare To Constant : simulink/Logic and Bit Operations/Compare To Constant  relop===  const=4900  OutDataTypeStr=boolean
  Compare To Constant1 : simulink/Logic and Bit Operations/Compare To Constant  relop===  const=1400  OutDataTypeStr=boolean
  Compare To Constant2 : simulink/Logic and Bit Operations/Compare To Constant  relop===  const=70  OutDataTypeStr=boolean
  Compare To Constant3 : simulink/Logic and Bit Operations/Compare To Constant  relop===  const=5000  OutDataTypeStr=boolean
  Compare To Constant4 : simulink/Logic and Bit Operations/Compare To Constant  relop===  const=4  OutDataTypeStr=boolean
  Compare To Constant5 : simulink/Logic and Bit Operations/Compare To Constant  relop===  const=0  OutDataTypeStr=boolean
  Constant1 : Constant  OutDataTypeStr=boolean
  Constant2 : Constant  Value=0  OutDataTypeStr=boolean
  Constant3 : Constant  Value=0  OutDataTypeStr=boolean
  Constant4 : Constant  OutDataTypeStr=uint8
  Constant5 : Constant  Value=0  OutDataTypeStr=uint8
  Constant6 : Constant  Value=2  OutDataTypeStr=uint8
  Constant7 : Constant  Value=0  OutDataTypeStr=uint8
  Data Type Conversion{1..5} (5 alike) : DataTypeConversion  OutDataTypeStr=boolean
  Data Type Conversion6 : DataTypeConversion  OutDataTypeStr=uint8
  Delay : Delay  DelayLength=1  InitialCondition=0
  Delay1 : Delay  DelayLength=1  InitialCondition=0
  Delay2 : Delay  InitialCondition=0
  Delay3 : Delay  DelayLength=1  InitialCondition=0
  HDL Counter : hdlsllib/HDL Operations/HDL Counter  CountType=Count limited  CountInit=0  CountStep=1  CountMax=6  CountFromType=Initial value  CountFrom=0  CountResetPort=on  CountLoadPort=off  CountEnbPort=on  CountDirPort=off  CountDataType=Unsigned  CountWordLen=3  CountFracLen=0  CountSampTime=277e-9
  HDL Counter1 : hdlsllib/HDL Operations/HDL Counter  CountType=Count limited  CountInit=0  CountStep=1  CountMax=40000  CountFromType=Initial value  CountFrom=0  CountResetPort=on  CountLoadPort=off  CountEnbPort=on  CountDirPort=off  CountDataType=Unsigned  CountWordLen=32  CountFracLen=0  CountSampTime=277e-9
  HDL Counter2 : hdlsllib/HDL Operations/HDL Counter  CountType=Free running  CountInit=0  CountStep=1  CountMax=6  CountFromType=Initial value  CountFrom=0  CountResetPort=off  CountLoadPort=off  CountEnbPort=on  CountDirPort=off  CountDataType=Unsigned  CountWordLen=1  CountFracLen=0  CountSampTime=277e-9
  Logical Operator : Logic  Operator=XOR  AllPortsSameDT=off  OutDataTypeStr=boolean
  Logical Operator{1,17..22} (7 alike) : Logic  Operator=OR  AllPortsSameDT=off  OutDataTypeStr=boolean
  Logical Operator{2,4..10,23} (9 alike) : Logic  AllPortsSameDT=off  OutDataTypeStr=boolean
  Logical Operator{3,11..15} (6 alike) : Logic  Operator=NOT  AllPortsSameDT=off  OutDataTypeStr=boolean
  Logical Operator16 : Logic  Operator=XOR  AllPortsSameDT=off  OutDataTypeStr=boolean
  SA{1..7} (7 alike) : simulink/Additional Math & Discrete/Additional Discrete/Unit Delay Enabled  vinit=0  tsamp=-1
  Switch{1..8} (8 alike) : Switch  Criteria=u2 ~= 0
  DataOUT : Outport  OutDataTypeStr=uint8
  Signal : Outport  Port=2  OutDataTypeStr=uint8
  ADR_OUT : Outport  Port=3  OutDataTypeStr=uint8
  wires:
  Addr/1 -> Compare To Constant4/1
  Data/1 -> Switch1/1
  Bit Concat1/1 -> Data Type Conversion6/1
  Bit Slice/1 -> Data Type Conversion2/1
  Bit Slice1/1 -> Data Type Conversion3/1
  Bit Slice2/1 -> Data Type Conversion4/1
  Bit Slice3/1 -> Data Type Conversion5/1
  Compare To Constant/1 -> Switch3/3, Logical Operator19/1
  Compare To Constant1/1 -> Switch4/3, Logical Operator20/2
  Compare To Constant2/1 -> Switch5/3, Logical Operator21/1
  Compare To Constant3/1 -> Switch6/3, Logical Operator22/2
  Compare To Constant4/1 -> Switch1/2
  Compare To Constant5/1 -> HDL Counter2/1
  Constant1/1 -> Delay2/1
  Constant2/1 -> Switch2/1
  Constant3/1 -> Switch6/1, Switch5/1, Switch4/1, Switch3/1
  Constant4/1 -> Switch7/1
  Constant5/1 -> Switch7/3
  Constant6/1 -> Switch8/1
  Constant7/1 -> Switch8/3
  Data Type Conversion1/1 -> Logical Operator7/1
  Data Type Conversion2/1 -> Logical Operator2/1, Logical Operator1/1
  Data Type Conversion3/1 -> Logical Operator3/1, Logical Operator1/2
  Data Type Conversion4/1 -> Logical Operator9/1, Logical Operator8/1, Logical Operator6/1, Logical Operator5/2, Logical Operator4/2
  Data Type Conversion5/1 -> Switch6/2, Switch5/2, Switch4/2, Switch3/2, Switch2/2, Logical Operator22/1, Logical Operator21/2, Logical Operator20/1, Logical Operator19/2, Logical Operator18/2, Logical Operator17/2
  Data Type Conversion6/1 -> Signal/1
  Delay/1 -> Logical Operator/2, Delay1/1
  Delay1/1 -> HDL Counter/2
  Delay2/1 -> Logical Operator10/1
  Delay3/1 -> Logical Operator16/1
  HDL Counter/1 -> Compare To Constant5/1
  HDL Counter1/1 -> Compare To Constant3/1, Compare To Constant2/1, Compare To Constant1/1, Compare To Constant/1
  HDL Counter2/1 -> Data Type Conversion1/1
  Logical Operator/1 -> Logical Operator17/1
  Logical Operator1/1 -> Logical Operator18/1
  Logical Operator10/1 -> HDL Counter1/2
  Logical Operator11/1 -> Logical Operator10/2
  Logical Operator12/1 -> Bit Concat1/1
  Logical Operator13/1 -> Logical Operator7/2
  Logical Operator14/1 -> Bit Concat1/3
  Logical Operator15/1 -> Bit Concat1/2
  Logical Operator16/1 -> Logical Operator23/1
  Logical Operator17/1 -> HDL Counter1/1, HDL Counter/1
  Logical Operator18/1 -> SA1/2
  Logical Operator19/1 -> SA3/2, SA2/2
  Logical Operator2/1 -> Switch2/3
  Logical Operator20/1 -> SA4/2
  Logical Operator21/1 -> SA5/2
  Logical Operator22/1 -> SA6/2
  Logical Operator23/1 -> Switch8/2
  Logical Operator3/1 -> Logical Operator2/2
  Logical Operator4/1 -> Logical Operator14/1
  Logical Operator5/1 -> Logical Operator15/1
  Logical Operator6/1 -> Logical Operator13/1
  Logical Operator7/1 -> Bit Concat1/4
  Logical Operator8/1 -> Logical Operator12/1
  Logical Operator9/1 -> Switch7/2, Logical Operator23/2, Logical Operator16/2, Logical Operator11/1, Delay3/1
  SA1/1 -> Logical Operator/1, Delay/1
  SA2/1 -> Logical Operator4/1
  SA3/1 -> Logical Operator5/1
  SA4/1 -> Logical Operator6/2
  SA5/1 -> Logical Operator8/2
  SA6/1 -> Logical Operator9/2
  SA7/1 -> Switch1/3, Bit Slice3/1, Bit Slice2/1, Bit Slice1/1, Bit Slice/1
  Switch1/1 -> SA7/2, SA7/1
  Switch2/1 -> SA1/1
  Switch3/1 -> SA3/1, SA2/1
  Switch4/1 -> SA4/1
  Switch5/1 -> SA5/1
  Switch6/1 -> SA6/1
  Switch7/1 -> DataOUT/1
  Switch8/1 -> ADR_OUT/1

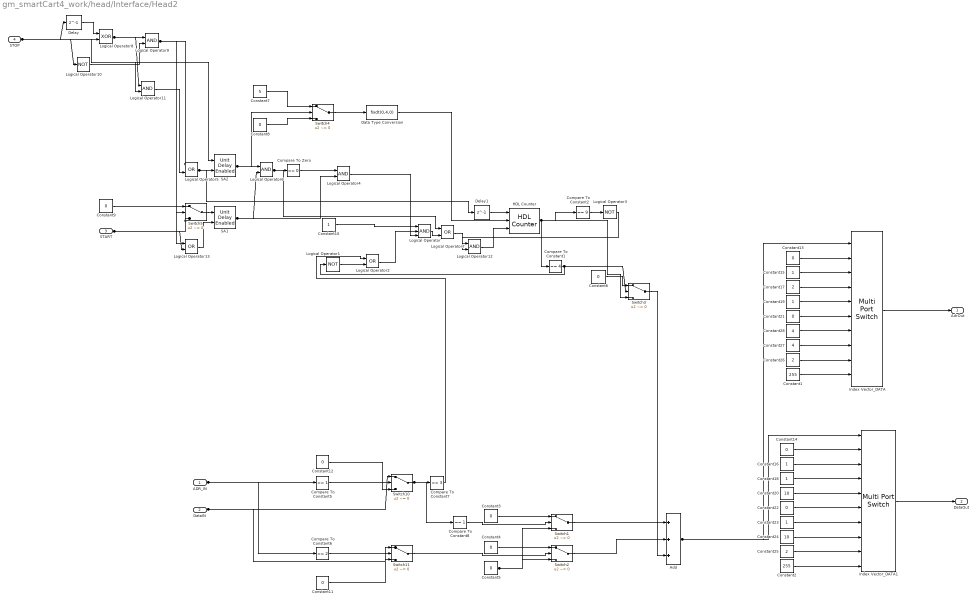
== system gm_smartCart4_work/head/Interface/Head2 ==
  ADR_IN : Inport  OutDataTypeStr=uint8  SampleTime=1
  DataIN : Inport  Port=2  OutDataTypeStr=uint8  SampleTime=1
  START : Inport  Port=3  OutDataTypeStr=boolean  SampleTime=1
  STOP : Inport  Port=4  OutDataTypeStr=boolean  SampleTime=1
  Add : Sum  Inputs=+++
  Compare To Constant1 : simulink/Logic and Bit Operations/Compare To Constant  relop===  const=4  OutDataTypeStr=boolean
  Compare To Constant2 : simulink/Logic and Bit Operations/Compare To Constant  relop===  const=9  OutDataTypeStr=boolean
  Compare To Constant5 : simulink/Logic and Bit Operations/Compare To Constant  relop===  const=1  OutDataTypeStr=boolean
  Compare To Constant6 : simulink/Logic and Bit Operations/Compare To Constant  relop===  const=2  OutDataTypeStr=boolean
  Compare To Constant7 : simulink/Logic and Bit Operations/Compare To Constant  relop===  const=3  OutDataTypeStr=boolean
  Compare To Constant8 : simulink/Logic and Bit Operations/Compare To Constant  relop===  const=1  OutDataTypeStr=boolean
  Compare To Zero : simulink/Logic and Bit Operations/Compare To Zero  relop===  OutDataTypeStr=boolean
  Constant1 : Constant  Value=255  OutDataTypeStr=uint8
  Constant10 : Constant  OutDataTypeStr=boolean
  Constant{3..6,11..14,21..22} (10 alike) : Constant  Value=0  OutDataTypeStr=uint8
  Constant{15..16,18..19,23} (5 alike) : Constant  OutDataTypeStr=uint8
  Constant17 : Constant  Value=2  OutDataTypeStr=uint8
  Constant2 : Constant  Value=255  OutDataTypeStr=uint8
  Constant20 : Constant  Value=10  OutDataTypeStr=uint8
  Constant24 : Constant  Value=10  OutDataTypeStr=uint8
  Constant25 : Constant  Value=2  OutDataTypeStr=uint8
  Constant26 : Constant  Value=2  OutDataTypeStr=uint8
  Constant27 : Constant  Value=4  OutDataTypeStr=uint8
  Constant28 : Constant  Value=4  OutDataTypeStr=uint8
  Constant7 : Constant  Value=5  OutDataTypeStr=fixdt(0,4,0)
  Constant8 : Constant  Value=0  OutDataTypeStr=fixdt(0,4,0)
  Constant9 : Constant  Value=0  OutDataTypeStr=boolean
  Data Type Conversion : DataTypeConversion  OutDataTypeStr=fixdt(0,4,0)
  Delay : Delay  DelayLength=1  InitialCondition=0
  Delay1 : Delay  DelayLength=1  InitialCondition=0
  HDL Counter : hdlsllib/HDL Operations/HDL Counter  CountType=Free running  CountInit=0  CountStep=1  CountMax=100  CountFromType=Initial value  CountFrom=0  CountResetPort=off  CountLoadPort=on  CountEnbPort=on  CountDirPort=off  CountDataType=Unsigned  CountWordLen=4  CountFracLen=0  CountSampTime=1
  Index Vector_DATA : MultiPortSwitch  DataPortOrder=Zero-based contiguous  Inputs=9  DiagnosticForDefault=None  zeroidx=on  OutDataTypeStr=uint8
  Index Vector_DATA1 : MultiPortSwitch  DataPortOrder=Zero-based contiguous  Inputs=9  DiagnosticForDefault=None  zeroidx=on  OutDataTypeStr=uint8
  Logical Operator : Logic  Inputs=3  AllPortsSameDT=off  OutDataTypeStr=boolean
  Logical Operator1 : Logic  Operator=NOT  AllPortsSameDT=off  OutDataTypeStr=boolean
  Logical Operator10 : Logic  Operator=NOT  AllPortsSameDT=off  OutDataTypeStr=boolean
  Logical Operator{4,6,9,11..12} (5 alike) : Logic  AllPortsSameDT=off  OutDataTypeStr=boolean
  Logical Operator{2,5,7,13} (4 alike) : Logic  Operator=OR  AllPortsSameDT=off  OutDataTypeStr=boolean
  Logical Operator3 : Logic  Operator=NOT  AllPortsSameDT=off  OutDataTypeStr=boolean
  Logical Operator8 : Logic  Operator=XOR  AllPortsSameDT=off  OutDataTypeStr=boolean
  SA1 : simulink/Additional Math & Discrete/Additional Discrete/Unit Delay Enabled  vinit=0  tsamp=-1
  SA2 : simulink/Additional Math & Discrete/Additional Discrete/Unit Delay Enabled  vinit=0  tsamp=-1
  Switch{1..5,10..11} (7 alike) : Switch  Criteria=u2 ~= 0  OutDataTypeStr=uint8
  AdrOut : Outport  OutDataTypeStr=uint8
  DataOut : Outport  Port=2  OutDataTypeStr=uint8
  wires:
  ADR_IN/1 -> Compare To Constant6/1, Compare To Constant5/1
  DataIN/1 -> Switch11/1, Switch10/1
  START/1 -> Switch5/3, Logical Operator13/2
  STOP/1 -> Logical Operator8/2, Logical Operator11/2, Logical Operator10/1, SA2/1, Delay/1
  Add/1 -> Index Vector_DATA1/1, Index Vector_DATA/1
  Compare To Constant1/1 -> Switch3/2, Logical Operator1/1
  Compare To Constant2/1 -> Logical Operator3/1
  Compare To Constant5/1 -> Switch10/2
  Compare To Constant6/1 -> Switch11/2
  Compare To Constant7/1 -> Logical Operator2/1
  Compare To Constant8/1 -> Switch1/2
  Compare To Zero/1 -> Logical Operator4/1
  Constant1/1 -> Index Vector_DATA/10
  Constant10/1 -> Logical Operator/1
  Constant11/1 -> Switch11/3
  Constant12/1 -> Switch10/3
  Constant13/1 -> Index Vector_DATA/2
  Constant14/1 -> Index Vector_DATA1/2
  Constant15/1 -> Index Vector_DATA/3
  Constant16/1 -> Index Vector_DATA1/3
  Constant17/1 -> Index Vector_DATA/4
  Constant18/1 -> Index Vector_DATA1/4
  Constant19/1 -> Index Vector_DATA/5
  Constant2/1 -> Index Vector_DATA1/10
  Constant20/1 -> Index Vector_DATA1/5
  Constant21/1 -> Index Vector_DATA/6
  Constant22/1 -> Index Vector_DATA1/6
  Constant23/1 -> Index Vector_DATA1/7
  Constant24/1 -> Index Vector_DATA1/8
  Constant25/1 -> Index Vector_DATA1/9
  Constant26/1 -> Index Vector_DATA/9
  Constant27/1 -> Index Vector_DATA/8
  Constant28/1 -> Index Vector_DATA/7
  Constant3/1 -> Switch1/1
  Constant4/1 -> Switch2/1
  Constant5/1 -> Switch2/3, Switch1/3
  Constant6/1 -> Switch3/1
  Constant7/1 -> Switch4/1
  Constant8/1 -> Switch4/3
  Constant9/1 -> Switch5/1
  Data Type Conversion/1 -> HDL Counter/2
  Delay/1 -> Logical Operator8/1
  Delay1/1 -> HDL Counter/1
  HDL Counter/1 -> Switch3/3, Compare To Constant2/1, Compare To Constant1/1
  Index Vector_DATA/1 -> AdrOut/1
  Index Vector_DATA1/1 -> DataOut/1
  Logical Operator/1 -> Logical Operator7/2
  Logical Operator1/1 -> Logical Operator2/2
  Logical Operator10/1 -> Logical Operator9/2
  Logical Operator11/1 -> Logical Operator5/2
  Logical Operator12/1 -> HDL Counter/3
  Logical Operator13/1 -> SA1/2
  Logical Operator2/1 -> Logical Operator/2
  Logical Operator3/1 -> Logical Operator12/2
  Logical Operator4/1 -> Logical Operator/3
  Logical Operator5/1 -> SA2/2, Delay1/1
  Logical Operator6/1 -> Logical Operator7/1, Compare To Zero/1
  Logical Operator7/1 -> Logical Operator12/1
  Logical Operator8/1 -> Logical Operator9/1, Logical Operator11/1
  Logical Operator9/1 -> Switch5/2, Logical Operator5/1, Logical Operator13/1
  SA1/1 -> Logical Operator6/2, Logical Operator4/2
  SA2/1 -> Switch4/2, Logical Operator6/1
  Switch1/1 -> Add/1
  Switch10/1 -> Compare To Constant8/1, Compare To Constant7/1
  Switch11/1 -> Switch2/2
  Switch2/1 -> Add/2
  Switch3/1 -> Add/3
  Switch4/1 -> Data Type Conversion/1
  Switch5/1 -> SA1/1
